simulink model "kopter_se_zavazim_simulace"  (R2024b)
settings: Solver=FixedStepAuto  StartTime=0.0  StopTime=5  FixedStep=0.01  RelTol=1e-3
values from neighbouring files (symbols this model uses):
  b_moment = 0.01    [parametry_kopter_se_zavazim.m]
  d = 1    [parametry_kopter_se_zavazim.m]
  g = 9.81    [parametry_kopter_se_zavazim.m]
  Ip = m*d^2    (= 1)    [parametry_kopter_se_zavazim.m]
  Ixx = 1.1    [parametry_kopter_se_zavazim.m]
  Iyy = 2.989    [parametry_kopter_se_zavazim.m]
  Izz = 3.978    [parametry_kopter_se_zavazim.m]
  k = 0.01    [parametry_kopter_se_zavazim.m]
  k_thrust = 0.1    [parametry_kopter_se_zavazim.m]
  L = 0.086    [parametry_kopter_se_zavazim.m]
  M = 3.3    [parametry_kopter_se_zavazim.m]
  m = 1    [parametry_kopter_se_zavazim.m]
  Us = [M*g; 0; 0; 0]    [parametry_kopter_se_zavazim.m]
  Xinit_matrix = [xyz_init; uhly_init; zavazi_init]    [parametry_kopter_se_zavazim.m]
  Xs = [0;0;0; 0;0;0; 0;0; 0;0;0; 0;0;0; 0;0]    [parametry_kopter_se_zavazim.m]
undefined symbols (not defined in the file or in its folder): Xinit_ss
libraries: simulink_extras x4
settings Model: Creator=Admin  LastModifiedBy=Admin

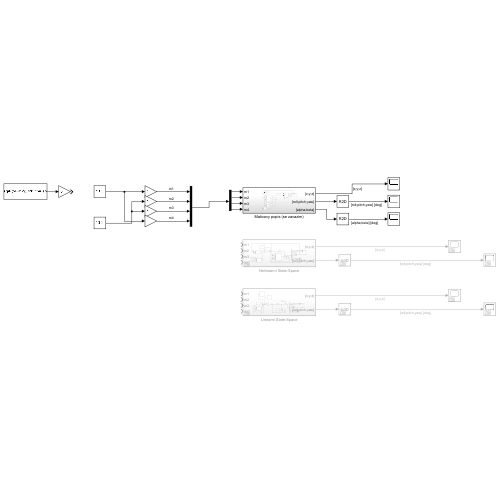
[thumbnail: Simulink's stored preview of the top-level diagram]
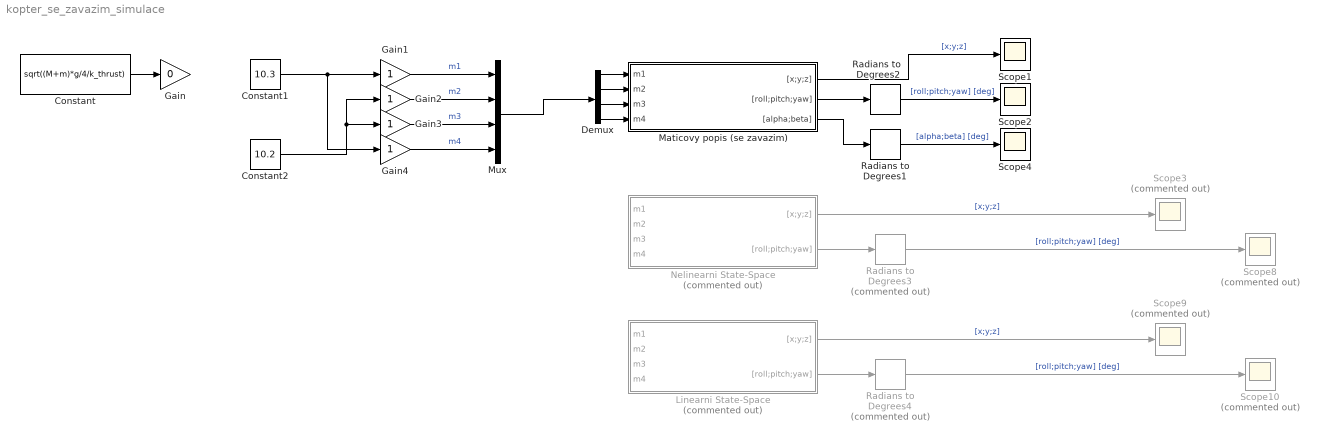
== system kopter_se_zavazim_simulace ==
  Constant : Constant  Value=sqrt((M+m)*g/4/k_thrust)
  Constant1 : Constant  Value=10.3
  Constant2 : Constant  Value=10.2
  Demux : Demux
  Gain : Gain  Gain=0
  Gain{1..4} (4 alike) : Gain
  Linearni State-Space : Subsystem  Commented=on
  Maticovy popis (se zavazim) : Subsystem
  Mux : Mux
  Nelinearni State-Space : Subsystem  Commented=on
  Radians to Degrees1 : simulink_extras/Transformations/Radians to Degrees
  Radians to Degrees2 : simulink_extras/Transformations/Radians to Degrees
  Radians to Degrees3 : simulink_extras/Transformations/Radians to Degrees  Commented=on
  Radians to Degrees4 : simulink_extras/Transformations/Radians to Degrees  Commented=on
  Scope1 : Scope
  Scope{3,8..10} (4 alike) : Scope  Commented=on
  Scope2 : Scope
  Scope4 : Scope
  wires:
  Gain4/1 -> Mux/4  "m4"
  Constant/1 -> Gain/1
  Gain1/1 -> Mux/1  "m1"
  Gain3/1 -> Mux/3  "m3"
  Gain2/1 -> Mux/2  "m2"
  Maticovy popis (se zavazim)/1("[x;y;z]") -> Scope1/1  "[x;y;z]"
  Radians to Degrees2/1 -> Scope2/1  "[roll;pitch;yaw] [deg]"
  Maticovy popis (se zavazim)/2("[roll;pitch;yaw]") -> Radians to Degrees2/1
  Radians to Degrees3/1 -> Scope8/1  "[roll;pitch;yaw] [deg]"
  Nelinearni State-Space/1("[x;y;z]") -> Scope3/1  "[x;y;z]"
  Nelinearni State-Space/2("[roll;pitch;yaw]") -> Radians to Degrees3/1
  Radians to Degrees4/1 -> Scope10/1  "[roll;pitch;yaw] [deg]"
  Linearni State-Space/2("[roll;pitch;yaw]") -> Radians to Degrees4/1
  Linearni State-Space/1("[x;y;z]") -> Scope9/1  "[x;y;z]"
  Constant1/1 -> Gain4/1, Gain1/1
  Constant2/1 -> Gain3/1, Gain2/1
  Maticovy popis (se zavazim)/3("[alpha;beta]") -> Radians to Degrees1/1
  Radians to Degrees1/1 -> Scope4/1  "[alpha;beta] [deg]"
  Demux/1 -> Maticovy popis (se zavazim)/1(m1)
  Demux/2 -> Maticovy popis (se zavazim)/2(m2)
  Demux/3 -> Maticovy popis (se zavazim)/3(m3)
  Demux/4 -> Maticovy popis (se zavazim)/4(m4)
  Mux/1 -> Demux/1

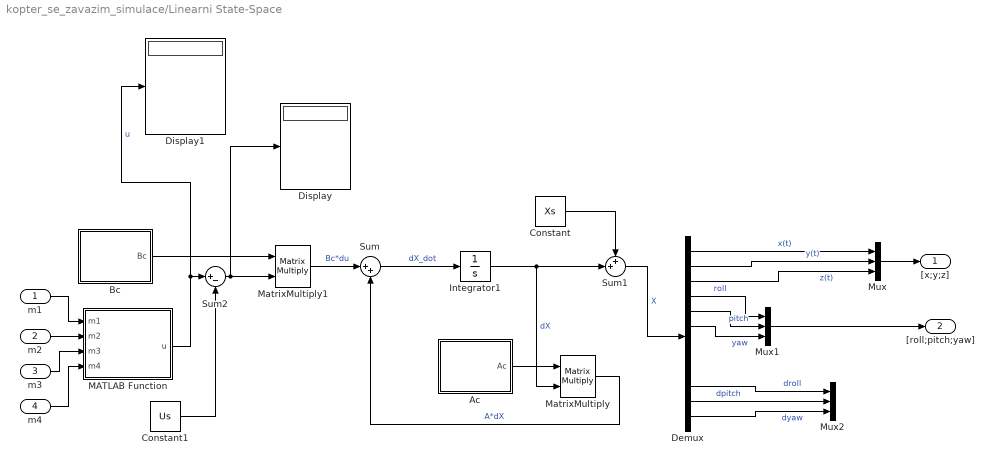
== system kopter_se_zavazim_simulace/Linearni State-Space ==
  m1 : Inport
  m2 : Inport  Port=2
  m3 : Inport  Port=3
  m4 : Inport  Port=4
  Ac : MATLAB Function  TreatAsAtomicUnit=on
  Bc : MATLAB Function  TreatAsAtomicUnit=on
  Constant : Constant  Value=Xs
  Constant1 : Constant  Value=Us
  Demux : Demux  Outputs=12
  Display : Display
  Display1 : Display
  Integrator1 : Integrator  InitialCondition=Xinit_ss
  MATLAB Function : MATLAB Function  TreatAsAtomicUnit=on
  MatrixMultiply : Product  Multiplication=Matrix(*)
  MatrixMultiply1 : Product  Multiplication=Matrix(*)
  Mux : Mux  Inputs=3
  Mux1 : Mux  Inputs=3
  Mux2 : Mux  Inputs=3
  Sum : Sum  Inputs=|++
  Sum1 : Sum  Inputs=++|
  Sum2 : Sum  Inputs=|+-
  "[x;y;z]" : Outport
  "[roll;pitch;yaw]" : Outport  Port=2
  wires:
  MATLAB Function/1(u) -> Display1/1, Sum2/1  "u"
  m3/1 -> MATLAB Function/3(m3)
  m2/1 -> MATLAB Function/2(m2)
  m4/1 -> MATLAB Function/4(m4)
  m1/1 -> MATLAB Function/1(m1)
  Ac/1(Ac) -> MatrixMultiply/1
  Integrator1/1 -> Sum1/2, MatrixMultiply/2  "dX"
  Demux/1 -> Mux/1  "x(t)"
  Demux/2 -> Mux/2  "y(t)"
  Demux/3 -> Mux/3  "z(t)"
  Mux/1 -> "[x;y;z]"/1
  Demux/4 -> Mux1/1  "roll"
  Demux/5 -> Mux1/2  "pitch"
  Demux/6 -> Mux1/3  "yaw"
  Mux1/1 -> "[roll;pitch;yaw]"/1
  Demux/10 -> Mux2/1  "droll"
  Demux/11 -> Mux2/2  "dpitch"
  Demux/12 -> Mux2/3  "dyaw"
  Sum/1 -> Integrator1/1  "dX_dot"
  MatrixMultiply1/1 -> Sum/1  "Bc*du"
  MatrixMultiply/1 -> Sum/2  "A*dX"
  Bc/1(Bc) -> MatrixMultiply1/1
  Sum1/1 -> Demux/1  "X"
  Constant/1 -> Sum1/1
  Constant1/1 -> Sum2/2
  Sum2/1 -> Display/1, MatrixMultiply1/2

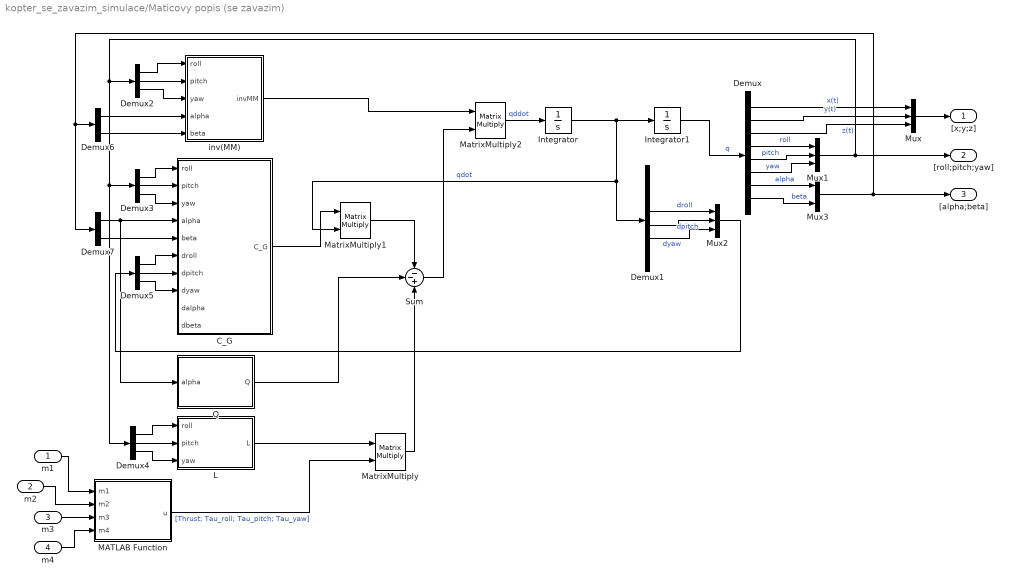
== system kopter_se_zavazim_simulace/Maticovy popis (se zavazim) ==
  m1 : Inport
  m2 : Inport  Port=2
  m3 : Inport  Port=3
  m4 : Inport  Port=4
  C_G : MATLAB Function  TreatAsAtomicUnit=on
  Demux : Demux  Outputs=8
  Demux1 : Demux  Outputs=8
  Demux{2..5} (4 alike) : Demux  Outputs=3
  Demux6 : Demux  Outputs=2
  Demux7 : Demux  Outputs=2
  Integrator : Integrator  InitialCondition=[0;0;0;0;0;0;0;0]
  Integrator1 : Integrator  InitialCondition=Xinit_matrix
  L : MATLAB Function  TreatAsAtomicUnit=on
  MATLAB Function : MATLAB Function  TreatAsAtomicUnit=on
  MatrixMultiply : Product  Multiplication=Matrix(*)
  MatrixMultiply1 : Product  Multiplication=Matrix(*)
  MatrixMultiply2 : Product  Multiplication=Matrix(*)
  Mux : Mux  Inputs=3
  Mux1 : Mux  Inputs=3
  Mux2 : Mux  Inputs=3
  Mux3 : Mux  Inputs=2
  Q : MATLAB Function  TreatAsAtomicUnit=on
  Sum : Sum  Inputs=--+
  inv(MM) : MATLAB Function  TreatAsAtomicUnit=on
  "[x;y;z]" : Outport
  "[roll;pitch;yaw]" : Outport  Port=2
  "[alpha;beta]" : Outport  Port=3
  wires:
  inv(MM)/1(invMM) -> MatrixMultiply2/1
  L/1(L) -> MatrixMultiply/1
  MATLAB Function/1(u) -> MatrixMultiply/2  "[Thrust; Tau_roll; Tau_pitch; Tau_yaw]"
  m3/1 -> MATLAB Function/3(m3)
  m2/1 -> MATLAB Function/2(m2)
  m4/1 -> MATLAB Function/4(m4)
  MatrixMultiply/1 -> Sum/3
  m1/1 -> MATLAB Function/1(m1)
  Q/1(Q) -> Sum/2
  C_G/1(C_G) -> MatrixMultiply1/1
  MatrixMultiply1/1 -> Sum/1
  Sum/1 -> MatrixMultiply2/2
  MatrixMultiply2/1 -> Integrator/1  "qddot"
  Integrator/1 -> MatrixMultiply1/2, Demux1/1, Integrator1/1  "qdot"
  Integrator1/1 -> Demux/1  "q"
  Demux/1 -> Mux/1  "x(t)"
  Demux/2 -> Mux/2  "y(t)"
  Demux/3 -> Mux/3  "z(t)"
  Mux/1 -> "[x;y;z]"/1
  Demux/4 -> Mux1/1  "roll"
  Demux/5 -> Mux1/2  "pitch"
  Demux/6 -> Mux1/3  "yaw"
  Mux1/1 -> "[roll;pitch;yaw]"/1, Demux4/1, Demux3/1, Demux2/1
  Demux1/4 -> Mux2/1  "droll"
  Demux1/5 -> Mux2/2  "dpitch"
  Demux1/6 -> Mux2/3  "dyaw"
  Demux2/1 -> inv(MM)/1(roll)
  Demux2/2 -> inv(MM)/2(pitch)
  Demux2/3 -> inv(MM)/3(yaw)
  Demux3/2 -> C_G/2(pitch)
  Demux3/1 -> C_G/1(roll)
  Demux3/3 -> C_G/3(yaw)
  Demux4/2 -> L/2(pitch)
  Demux4/1 -> L/1(roll)
  Demux4/3 -> L/3(yaw)
  Demux5/2 -> C_G/7(dpitch)
  Demux5/1 -> C_G/6(droll)
  Demux5/3 -> C_G/8(dyaw)
  Mux2/1 -> Demux5/1
  Demux/7 -> Mux3/1  "alpha"
  Demux/8 -> Mux3/2  "beta"
  Mux3/1 -> Demux7/1, Demux6/1, "[alpha;beta]"/1
  Demux6/1 -> inv(MM)/4(alpha)
  Demux6/2 -> inv(MM)/5(beta)
  Demux7/2 -> C_G/5(beta)
  Demux7/1 -> Q/1(alpha), C_G/4(alpha)

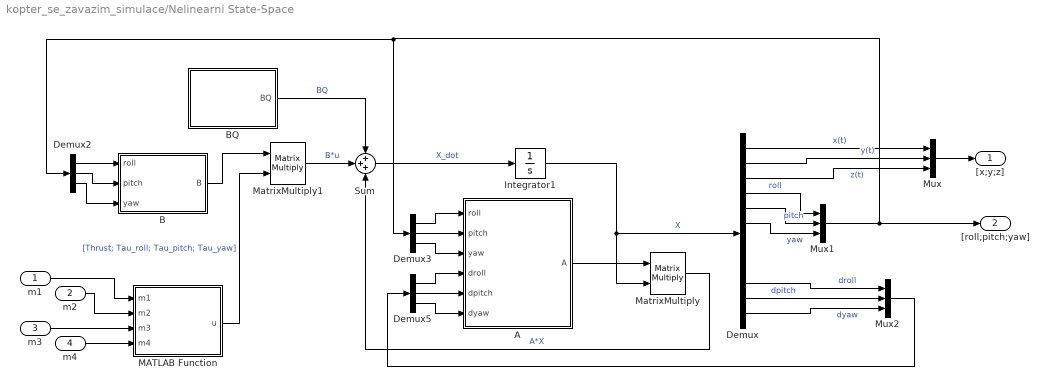
== system kopter_se_zavazim_simulace/Nelinearni State-Space ==
  m1 : Inport
  m2 : Inport  Port=2
  m3 : Inport  Port=3
  m4 : Inport  Port=4
  A : MATLAB Function  TreatAsAtomicUnit=on
  B : MATLAB Function  TreatAsAtomicUnit=on
  BQ : MATLAB Function  TreatAsAtomicUnit=on
  Demux : Demux  Outputs=12
  Demux2 : Demux  Outputs=3
  Demux3 : Demux  Outputs=3
  Demux5 : Demux  Outputs=3
  Integrator1 : Integrator  InitialCondition=Xinit_ss
  MATLAB Function : MATLAB Function  TreatAsAtomicUnit=on
  MatrixMultiply : Product  Multiplication=Matrix(*)
  MatrixMultiply1 : Product  Multiplication=Matrix(*)
  Mux : Mux  Inputs=3
  Mux1 : Mux  Inputs=3
  Mux2 : Mux  Inputs=3
  Sum : Sum  Inputs=+++
  "[x;y;z]" : Outport
  "[roll;pitch;yaw]" : Outport  Port=2
  wires:
  MATLAB Function/1(u) -> MatrixMultiply1/2  "[Thrust; Tau_roll; Tau_pitch; Tau_yaw]"
  m3/1 -> MATLAB Function/3(m3)
  m2/1 -> MATLAB Function/2(m2)
  m4/1 -> MATLAB Function/4(m4)
  m1/1 -> MATLAB Function/1(m1)
  A/1(A) -> MatrixMultiply/1
  Integrator1/1 -> Demux/1, MatrixMultiply/2  "X"
  Demux/1 -> Mux/1  "x(t)"
  Demux/2 -> Mux/2  "y(t)"
  Demux/3 -> Mux/3  "z(t)"
  Mux/1 -> "[x;y;z]"/1
  Demux/4 -> Mux1/1  "roll"
  Demux/5 -> Mux1/2  "pitch"
  Demux/6 -> Mux1/3  "yaw"
  Mux1/1 -> Demux2/1, Demux3/1, "[roll;pitch;yaw]"/1
  Demux/10 -> Mux2/1  "droll"
  Demux/11 -> Mux2/2  "dpitch"
  Demux/12 -> Mux2/3  "dyaw"
  Demux2/1 -> B/1(roll)
  Demux2/2 -> B/2(pitch)
  Demux2/3 -> B/3(yaw)
  Demux3/2 -> A/2(pitch)
  Demux3/1 -> A/1(roll)
  Demux3/3 -> A/3(yaw)
  Demux5/2 -> A/5(dpitch)
  Demux5/1 -> A/4(droll)
  Demux5/3 -> A/6(dyaw)
  Sum/1 -> Integrator1/1  "X_dot"
  BQ/1(BQ) -> Sum/1  "BQ"
  MatrixMultiply1/1 -> Sum/2  "B*u"
  B/1(B) -> MatrixMultiply1/1
  MatrixMultiply/1 -> Sum/3  "A*X"
  Mux2/1 -> Demux5/1

== matlab function kopter_se_zavazim_simulace/Nelinearni State-Space/BQ ==
  data: BQ output; g parameter
function BQ = fcn(g)
% Matice vstupu tihy
BQ = [0 0 0 0 0 0 0 0 -g 0 0 0]';

== matlab function kopter_se_zavazim_simulace/Nelinearni State-Space/MATLAB Function ==
  data: u output; m1 input; m2 input; m3 input; m4 input; k_thrust parameter; b_moment parameter; L parameter
function u = fcn(m1, m2, m3, m4, k_thrust, b_moment, L)

Thrust = k_thrust*(m1^2 + m2^2 + m3^2 + m4^2);
Tau_roll = L*k_thrust*(m1^2 + m4^2 - m2^2 - m3^2);
Tau_pitch = L*k_thrust*(m4^2 + m3^2 - m1^2 - m2^2);
Tau_yaw = b_moment*(m1^2 + m3^2 - m2^2 - m4^2);

u = [Thrust; Tau_roll; Tau_pitch; Tau_yaw];

== matlab function kopter_se_zavazim_simulace/Linearni State-Space/Bc ==
  data: M parameter; Bc output; Ixx parameter; Iyy parameter; Izz parameter
function Bc = fcn(M, Ixx, Iyy, Izz)
% Matice Ac linearizovana

Bc = [
  0,     0,     0,     0;
  0,     0,     0,     0;
  0,     0,     0,     0;
  0,     0,     0,     0;
  0,     0,     0,     0;
  0,     0,     0,     0;
  0,     0,     0,     0;
  0,     0,     0,     0;
1/M,     0,     0,     0;
  0, 1/Ixx,     0,     0;
  0,     0, 1/Iyy,     0;
  0,     0,     0, 1/Izz];

== matlab function kopter_se_zavazim_simulace/Nelinearni State-Space/B ==
  data: roll input; B output; pitch input; yaw input; M parameter; Ixx parameter; Iyy parameter; Izz parameter
function B = fcn(roll, pitch, yaw, M, Ixx, Iyy, Izz)
% Matice vstupu do soustavy kvadrokoptery

phi_t = roll;
theta_t = pitch;
psi_t = yaw;

B = [
                                                              0,     0,                                                                          0,                                                                          0;
                                                              0,     0,                                                                          0,                                                                          0;
                                                              0,     0,                                                                          0,                                                                          0;
                                                              0,     0,                                                                          0,                                                                          0;
                                                              0,     0,                                                                          0,                                                                          0;
                                                              0,     0,                                                                          0,                                                                          0;
 (sin(phi_t)*sin(psi_t) + cos(phi_t)*cos(psi_t)*sin(theta_t))/M,     0,                                                                          0,                                                                          0;
-(cos(psi_t)*sin(phi_t) - cos(phi_t)*sin(psi_t)*sin(theta_t))/M,     0,                                                                          0,                                                                          0;
                                    (cos(phi_t)*cos(theta_t))/M,     0,                                                                          0,                                                                          0;
                                                              0, 1/Ixx, (sin(phi_t)*sin(theta_t))/(Iyy*cos(theta_t)*(cos(phi_t)^2 + sin(phi_t)^2)), (cos(phi_t)*sin(theta_t))/(Izz*cos(theta_t)*(cos(phi_t)^2 + sin(phi_t)^2));
                                                              0,     0,                             cos(phi_t)/(Iyy*(cos(phi_t)^2 + sin(phi_t)^2)),                            -sin(phi_t)/(Izz*(cos(phi_t)^2 + sin(phi_t)^2));
                                                              0,     0,                sin(phi_t)/(Iyy*cos(theta_t)*(cos(phi_t)^2 + sin(phi_t)^2)),                cos(phi_t)/(Izz*cos(theta_t)*(cos(phi_t)^2 + sin(phi_t)^2))];

== matlab function kopter_se_zavazim_simulace/Linearni State-Space/MATLAB Function ==
  data: u output; m1 input; m2 input; m3 input; m4 input; k_thrust parameter; b_moment parameter; L parameter
function u = fcn(m1, m2, m3, m4, k_thrust, b_moment, L)

Thrust = k_thrust*(m1^2 + m2^2 + m3^2 + m4^2);
Tau_roll = L*k_thrust*(m1^2 + m4^2 - m2^2 - m3^2);
Tau_pitch = L*k_thrust*(m4^2 + m3^2 - m1^2 - m2^2);
Tau_yaw = b_moment*(m1^2 + m3^2 - m2^2 - m4^2);

u = [Thrust; Tau_roll; Tau_pitch; Tau_yaw];

== matlab function kopter_se_zavazim_simulace/Linearni State-Space/Ac ==
  data: Ac output; k parameter; g parameter; M parameter
function Ac = fcn(k, g, M)
% Matice Ac linearizovana

Ac = [ 
0, 0, 0,  0, 0, 0,    1,    0,    0, 0, 0, 0;
0, 0, 0,  0, 0, 0,    0,    1,    0, 0, 0, 0;
0, 0, 0,  0, 0, 0,    0,    0,    1, 0, 0, 0;
0, 0, 0,  0, 0, 0,    0,    0,    0, 1, 0, 0;
0, 0, 0,  0, 0, 0,    0,    0,    0, 0, 1, 0;
0, 0, 0,  0, 0, 0,    0,    0,    0, 0, 0, 1;
0, 0, 0,  0, g, 0, -k/M,    0,    0, 0, 0, 0;
0, 0, 0, -g, 0, 0,    0, -k/M,    0, 0, 0, 0;
0, 0, 0,  0, 0, 0,    0,    0, -k/M, 0, 0, 0;
0, 0, 0,  0, 0, 0,    0,    0,    0, 0, 0, 0;
0, 0, 0,  0, 0, 0,    0,    0,    0, 0, 0, 0;
0, 0, 0,  0, 0, 0,    0,    0,    0, 0, 0, 0];

== matlab function kopter_se_zavazim_simulace/Maticovy popis (se zavazim)/C_G ==
  data: roll input; C_G output; pitch input; yaw input; alpha input; beta input; droll input; dpitch input; dyaw input; dalpha input; dbeta input; Ixx parameter; Iyy parameter; Izz parameter; d parameter; m parameter
function C_G = fcn(roll, pitch, yaw, alpha, beta, droll, dpitch, dyaw, dalpha, dbeta, Ixx, Iyy, Izz, d, m)
% Matice Coriolisovych sil a odporu vzduchu

phi_t = roll;
theta_t = pitch;
psi_t = yaw;

phi_dot_t = droll;
theta_dot_t = dpitch;
psi_dot_t = dyaw;

alpha_t = alpha;
beta_t = beta;

alpha_dot_t = dalpha;
beta_dot_t = dbeta;


C_G = [
0, 0, 0,                                                                                                                                                                                                                                                                    0,                                                                                                                                                                                                                                           0,                                                                                                                                   0,                                                         - alpha_dot_t*d*m*cos(beta_t)*sin(alpha_t) - 2*beta_dot_t*d*m*cos(alpha_t)*sin(beta_t),                                                                    -beta_dot_t*d*m*cos(beta_t)*sin(alpha_t);
0, 0, 0,                                                                                                                                                                                                                                                                    0,                                                                                                                                                                                                                                           0,                                                                                                                                   0,                                                           2*beta_dot_t*d*m*cos(alpha_t)*cos(beta_t) - alpha_dot_t*d*m*sin(alpha_t)*sin(beta_t),                                                                    -beta_dot_t*d*m*sin(alpha_t)*sin(beta_t);
0, 0, 0,                                                                                                                                                                                                                                                                    0,                                                                                                                                                                                                                                           0,                                                                                                                                   0,                                                                                                                   alpha_dot_t*d*m*cos(alpha_t),                                                                                                           0;
0, 0, 0,                                                                                                                                                                                                                                                                    0,          theta_dot_t*(Iyy*cos(phi_t)*sin(phi_t) - Izz*cos(phi_t)*sin(phi_t)) - psi_dot_t*(Ixx*cos(theta_t) + Iyy*cos(phi_t)^2*cos(theta_t) - Izz*cos(phi_t)^2*cos(theta_t) - Iyy*cos(theta_t)*sin(phi_t)^2 + Izz*cos(theta_t)*sin(phi_t)^2),                                    -psi_dot_t*(Iyy*cos(phi_t)*cos(theta_t)^2*sin(phi_t) - Izz*cos(phi_t)*cos(theta_t)^2*sin(phi_t)),                                                                                                                                              0,                                                                                                           0;
0, 0, 0,                               psi_dot_t*(Ixx*cos(theta_t) + Iyy*cos(phi_t)^2*cos(theta_t) - Izz*cos(phi_t)^2*cos(theta_t) - Iyy*cos(theta_t)*sin(phi_t)^2 + Izz*cos(theta_t)*sin(phi_t)^2) - theta_dot_t*(2*Iyy*cos(phi_t)*sin(phi_t) - 2*Izz*cos(phi_t)*sin(phi_t)),                                                                                                                                                                                                                                           0, psi_dot_t*(Izz*cos(phi_t)^2*cos(theta_t)*sin(theta_t) - Ixx*cos(theta_t)*sin(theta_t) + Iyy*cos(theta_t)*sin(phi_t)^2*sin(theta_t)),                                                                                                                                              0,                                                                                                           0;
0, 0, 0, psi_dot_t*(2*Iyy*cos(phi_t)*cos(theta_t)^2*sin(phi_t) - 2*Izz*cos(phi_t)*cos(theta_t)^2*sin(phi_t)) - theta_dot_t*(Ixx*cos(theta_t) - Iyy*cos(phi_t)^2*cos(theta_t) + Izz*cos(phi_t)^2*cos(theta_t) + Iyy*cos(theta_t)*sin(phi_t)^2 - Izz*cos(theta_t)*sin(phi_t)^2), - theta_dot_t*(Iyy*cos(phi_t)*sin(phi_t)*sin(theta_t) - Izz*cos(phi_t)*sin(phi_t)*sin(theta_t)) - psi_dot_t*(2*Izz*cos(phi_t)^2*cos(theta_t)*sin(theta_t) - 2*Ixx*cos(theta_t)*sin(theta_t) + 2*Iyy*cos(theta_t)*sin(phi_t)^2*sin(theta_t)),                                                                                                                                   0,                                                                                                                                              0,                                                                                                           0;
0, 0, 0,                                                                                                                                                                                                                                                                    0,                                                                                                                                                                                                                                           0,                                                                                                                                   0, -alpha_dot_t*(d^2*m*cos(alpha_t)*cos(beta_t)^2*sin(alpha_t) - d^2*m*cos(alpha_t)*sin(alpha_t) + d^2*m*cos(alpha_t)*sin(alpha_t)*sin(beta_t)^2), -beta_dot_t*(m*cos(alpha_t)*sin(alpha_t)*d^2*cos(beta_t)^2 + m*cos(alpha_t)*sin(alpha_t)*d^2*sin(beta_t)^2);
0, 0, 0,                                                                                                                                                                                                                                                                    0,                                                                                                                                                                                                                                           0,                                                                                                                                   0,                                 beta_dot_t*(2*d^2*m*cos(alpha_t)*cos(beta_t)^2*sin(alpha_t) + 2*d^2*m*cos(alpha_t)*sin(alpha_t)*sin(beta_t)^2),                                                                                                           0];

== matlab function kopter_se_zavazim_simulace/Maticovy popis (se zavazim)/inv(MM) ==
  data: roll input; invMM output; pitch input; yaw input; alpha input; beta input; M parameter; Ixx parameter; Iyy parameter; Izz parameter; d parameter; m parameter; Ip parameter
function invMM = fcn(roll, pitch, yaw, alpha, beta, M, Ixx, Iyy, Izz, d, m, Ip)
% Matice hmotnosti a setrvacnosti

phi_t = roll;
theta_t = pitch;
psi_t = yaw;

alpha_t = alpha;
beta_t = beta;

MM = [
                        M + m,                            0,                0,                 0,                                              0,                                                                                      0, d*m*cos(alpha_t)*cos(beta_t), -d*m*sin(alpha_t)*sin(beta_t);
                            0,                        M + m,                0,                 0,                                              0,                                                                                      0, d*m*cos(alpha_t)*sin(beta_t),  d*m*cos(beta_t)*sin(alpha_t);
                            0,                            0,            M + m,                 0,                                              0,                                                                                      0,             d*m*sin(alpha_t),                             0;
                            0,                            0,                0,               Ixx,                                              0,                                                                      -Ixx*sin(theta_t),                            0,                             0;
                            0,                            0,                0,                 0,      Iyy - Iyy*sin(phi_t)^2 + Izz*sin(phi_t)^2,                                         cos(phi_t)*cos(theta_t)*sin(phi_t)*(Iyy - Izz),                            0,                             0;
                            0,                            0,                0, -Ixx*sin(theta_t), cos(phi_t)*cos(theta_t)*sin(phi_t)*(Iyy - Izz), Izz*cos(phi_t)^2*cos(theta_t)^2 + Iyy*cos(theta_t)^2*sin(phi_t)^2 + Ixx*sin(theta_t)^2,                            0,                             0;
 d*m*cos(alpha_t)*cos(beta_t), d*m*cos(alpha_t)*sin(beta_t), d*m*sin(alpha_t),                 0,                                              0,                                                                                      0,                   m*d^2 + Ip,                             0;
-d*m*sin(alpha_t)*sin(beta_t), d*m*cos(beta_t)*sin(alpha_t),                0,                 0,                                              0,                                                                                      0,                            0,     m*d^2*sin(alpha_t)^2 + Ip];
 

invMM = inv(MM);

== matlab function kopter_se_zavazim_simulace/Maticovy popis (se zavazim)/Q ==
  data: alpha input; M parameter; Q output; g parameter; m parameter; d parameter
function Q = fcn(alpha, M, g, m, d)
alpha_t = alpha;
% Matice tihovych sil
Q = [0 0 (M+m)*g 0 0 0 d*g*m*sin(alpha_t) 0]';

== matlab function kopter_se_zavazim_simulace/Maticovy popis (se zavazim)/L ==
  data: roll input; L output; pitch input; yaw input
function L = fcn(roll, pitch, yaw)
% Matice vah vstupu

phi_t = roll;
theta_t = pitch;
psi_t = yaw;

L = [
sin(phi_t)*sin(psi_t) + cos(phi_t)*cos(psi_t)*sin(theta_t), 0, 0, 0;
cos(phi_t)*sin(psi_t)*sin(theta_t) - cos(psi_t)*sin(phi_t), 0, 0, 0;
                                   cos(phi_t)*cos(theta_t), 0, 0, 0;
                                                         0, 1, 0, 0;
                                                         0, 0, 1, 0;
                                                         0, 0, 0, 1;
                                                         0, 0, 0, 0;
                                                         0, 0, 0, 0];

== matlab function kopter_se_zavazim_simulace/Maticovy popis (se zavazim)/MATLAB Function ==
  data: u output; m1 input; m2 input; m3 input; m4 input; k_thrust parameter; b_moment parameter; L parameter
function u = fcn(m1, m2, m3, m4, k_thrust, b_moment, L)

Thrust = k_thrust*(m1^2 + m2^2 + m3^2 + m4^2);
Tau_roll = L*k_thrust*(m1^2 + m4^2 - m2^2 - m3^2);
Tau_pitch = L*k_thrust*(m4^2 + m3^2 - m1^2 - m2^2);
Tau_yaw = b_moment*(m1^2 + m3^2 - m2^2 - m4^2);

u = [Thrust; Tau_roll; Tau_pitch; Tau_yaw];

== matlab function kopter_se_zavazim_simulace/Nelinearni State-Space/A ==
  data: roll input; A output; pitch input; yaw input; droll input; dpitch input; dyaw input; k parameter; Ixx parameter; Iyy parameter; Izz parameter; M parameter
function A = fcn(roll, pitch, yaw, droll, dpitch, dyaw, k, Ixx, Iyy, Izz, M)
% Matice dynamiky A

phi_t = roll;
theta_t = pitch;
psi_t = yaw;

phi_dot_t = droll;
theta_dot_t = dpitch;
psi_dot_t = dyaw;

A = [
0, 0, 0, 0, 0, 0,    1,    0,    0,                                                                                                                                                                                                                                                                                                                                                                                                                                                                                                                               0,                                                                                                                                                                                                                                                                                                                                                                                                                                                                                                                                                                                                                                    0,                                                                                                                                                                                                                                                                                                                                                                                                                                                                                         0;
0, 0, 0, 0, 0, 0,    0,    1,    0,                                                                                                                                                                                                                                                                                                                                                                                                                                                                                                                               0,                                                                                                                                                                                                                                                                                                                                                                                                                                                                                                                                                                                                                                    0,                                                                                                                                                                                                                                                                                                                                                                                                                                                                                         0;
0, 0, 0, 0, 0, 0,    0,    0,    1,                                                                                                                                                                                                                                                                                                                                                                                                                                                                                                                               0,                                                                                                                                                                                                                                                                                                                                                                                                                                                                                                                                                                                                                                    0,                                                                                                                                                                                                                                                                                                                                                                                                                                                                                         0;
0, 0, 0, 0, 0, 0,    0,    0,    0,                                                                                                                                                                                                                                                                                                                                                                                                                                                                                                                               1,                                                                                                                                                                                                                                                                                                                                                                                                                                                                                                                                                                                                                                    0,                                                                                                                                                                                                                                                                                                                                                                                                                                                                                         0;
0, 0, 0, 0, 0, 0,    0,    0,    0,                                                                                                                                                                                                                                                                                                                                                                                                                                                                                                                               0,                                                                                                                                                                                                                                                                                                                                                                                                                                                                                                                                                                                                                                    1,                                                                                                                                                                                                                                                                                                                                                                                                                                                                                         0;
0, 0, 0, 0, 0, 0,    0,    0,    0,                                                                                                                                                                                                                                                                                                                                                                                                                                                                                                                               0,                                                                                                                                                                                                                                                                                                                                                                                                                                                                                                                                                                                                                                    0,                                                                                                                                                                                                                                                                                                                                                                                                                                                                                         1;
0, 0, 0, 0, 0, 0, -k/M,    0,    0,                                                                                                                                                                                                                                                                                                                                                                                                                                                                                                                               0,                                                                                                                                                                                                                                                                                                                                                                                                                                                                                                                                                                                                                                    0,                                                                                                                                                                                                                                                                                                                                                                                                                                                                                         0;
0, 0, 0, 0, 0, 0,    0, -k/M,    0,                                                                                                                                                                                                                                                                                                                                                                                                                                                                                                                               0,                                                                                                                                                                                                                                                                                                                                                                                                                                                                                                                                                                                                                                    0,                                                                                                                                                                                                                                                                                                                                                                                                                                                                                         0;
0, 0, 0, 0, 0, 0,    0,    0, -k/M,                                                                                                                                                                                                                                                                                                                                                                                                                                                                                                                               0,                                                                                                                                                                                                                                                                                                                                                                                                                                                                                                                                                                                                                                    0,                                                                                                                                                                                                                                                                                                                                                                                                                                                                                         0;
0, 0, 0, 0, 0, 0,    0,    0,    0, (cos(phi_t)*sin(theta_t)*(psi_dot_t*(Ixx*cos(theta_t)*sin(phi_t) - Iyy*cos(theta_t)*sin(phi_t) + Izz*cos(theta_t)*sin(phi_t)) + theta_dot_t*(Ixx*cos(phi_t) - Iyy*cos(phi_t) + Izz*cos(phi_t))))/(Izz*(cos(theta_t)*cos(phi_t)^2 + cos(theta_t)*sin(phi_t)^2)) - (sin(phi_t)*sin(theta_t)*(psi_dot_t*(Ixx*cos(phi_t)*cos(theta_t) + Iyy*cos(phi_t)*cos(theta_t) - Izz*cos(phi_t)*cos(theta_t)) - theta_dot_t*(Ixx*sin(phi_t) + Iyy*sin(phi_t) - Izz*sin(phi_t))))/(Iyy*(cos(theta_t)*cos(phi_t)^2 + cos(theta_t)*sin(phi_t)^2)), (psi_dot_t*(Ixx*cos(theta_t) + Iyy*cos(phi_t)^2*cos(theta_t) - Izz*cos(phi_t)^2*cos(theta_t) - Iyy*cos(theta_t)*sin(phi_t)^2 + Izz*cos(theta_t)*sin(phi_t)^2) - theta_dot_t*(Iyy*cos(phi_t)*sin(phi_t) - Izz*cos(phi_t)*sin(phi_t)))/Ixx + (psi_dot_t*cos(phi_t)*sin(theta_t)*(Iyy*cos(phi_t)*sin(theta_t) - Ixx*cos(phi_t)*sin(theta_t) + Izz*cos(phi_t)*sin(theta_t)))/(Izz*(cos(theta_t)*cos(phi_t)^2 + cos(theta_t)*sin(phi_t)^2)) + (psi_dot_t*sin(phi_t)*sin(theta_t)*(Iyy*sin(phi_t)*sin(theta_t) - Ixx*sin(phi_t)*sin(theta_t) + Izz*sin(phi_t)*sin(theta_t)))/(Iyy*(cos(theta_t)*cos(phi_t)^2 + cos(theta_t)*sin(phi_t)^2)), (psi_dot_t*(Iyy*cos(phi_t)*cos(theta_t)^2*sin(phi_t) - Izz*cos(phi_t)*cos(theta_t)^2*sin(phi_t)))/Ixx + (psi_dot_t*sin(phi_t)*sin(theta_t)*(Ixx*cos(phi_t)*cos(theta_t)*sin(theta_t) - Izz*cos(phi_t)*cos(theta_t)*sin(theta_t)))/(Iyy*(cos(theta_t)*cos(phi_t)^2 + cos(theta_t)*sin(phi_t)^2)) - (psi_dot_t*cos(phi_t)*sin(theta_t)*(Ixx*cos(theta_t)*sin(phi_t)*sin(theta_t) - Iyy*cos(theta_t)*sin(phi_t)*sin(theta_t)))/(Izz*(cos(theta_t)*cos(phi_t)^2 + cos(theta_t)*sin(phi_t)^2));
0, 0, 0, 0, 0, 0,    0,    0,    0,                                                                             - (cos(phi_t)*(psi_dot_t*(Ixx*cos(phi_t)*cos(theta_t) + Iyy*cos(phi_t)*cos(theta_t) - Izz*cos(phi_t)*cos(theta_t)) - theta_dot_t*(Ixx*sin(phi_t) + Iyy*sin(phi_t) - Izz*sin(phi_t))))/(Iyy*(cos(phi_t)^2 + sin(phi_t)^2)) - (sin(phi_t)*(psi_dot_t*(Ixx*cos(theta_t)*sin(phi_t) - Iyy*cos(theta_t)*sin(phi_t) + Izz*cos(theta_t)*sin(phi_t)) + theta_dot_t*(Ixx*cos(phi_t) - Iyy*cos(phi_t) + Izz*cos(phi_t))))/(Izz*(cos(phi_t)^2 + sin(phi_t)^2)),                                                                                                                                                                                                                                                                                                                          (psi_dot_t*cos(phi_t)*(Iyy*sin(phi_t)*sin(theta_t) - Ixx*sin(phi_t)*sin(theta_t) + Izz*sin(phi_t)*sin(theta_t)))/(Iyy*(cos(phi_t)^2 + sin(phi_t)^2)) - (psi_dot_t*sin(phi_t)*(Iyy*cos(phi_t)*sin(theta_t) - Ixx*cos(phi_t)*sin(theta_t) + Izz*cos(phi_t)*sin(theta_t)))/(Izz*(cos(phi_t)^2 + sin(phi_t)^2)),                                                                                                                                                                                       (psi_dot_t*cos(phi_t)*(Ixx*cos(phi_t)*cos(theta_t)*sin(theta_t) - Izz*cos(phi_t)*cos(theta_t)*sin(theta_t)))/(Iyy*(cos(phi_t)^2 + sin(phi_t)^2)) + (psi_dot_t*sin(phi_t)*(Ixx*cos(theta_t)*sin(phi_t)*sin(theta_t) - Iyy*cos(theta_t)*sin(phi_t)*sin(theta_t)))/(Izz*(cos(phi_t)^2 + sin(phi_t)^2));
0, 0, 0, 0, 0, 0,    0,    0,    0,                           (cos(phi_t)*(psi_dot_t*(Ixx*cos(theta_t)*sin(phi_t) - Iyy*cos(theta_t)*sin(phi_t) + Izz*cos(theta_t)*sin(phi_t)) + theta_dot_t*(Ixx*cos(phi_t) - Iyy*cos(phi_t) + Izz*cos(phi_t))))/(Izz*(cos(theta_t)*cos(phi_t)^2 + cos(theta_t)*sin(phi_t)^2)) - (sin(phi_t)*(psi_dot_t*(Ixx*cos(phi_t)*cos(theta_t) + Iyy*cos(phi_t)*cos(theta_t) - Izz*cos(phi_t)*cos(theta_t)) - theta_dot_t*(Ixx*sin(phi_t) + Iyy*sin(phi_t) - Izz*sin(phi_t))))/(Iyy*(cos(theta_t)*cos(phi_t)^2 + cos(theta_t)*sin(phi_t)^2)),                                                                                                                                                                                                                                                                      (psi_dot_t*cos(phi_t)*(Iyy*cos(phi_t)*sin(theta_t) - Ixx*cos(phi_t)*sin(theta_t) + Izz*cos(phi_t)*sin(theta_t)))/(Izz*(cos(theta_t)*cos(phi_t)^2 + cos(theta_t)*sin(phi_t)^2)) + (psi_dot_t*sin(phi_t)*(Iyy*sin(phi_t)*sin(theta_t) - Ixx*sin(phi_t)*sin(theta_t) + Izz*sin(phi_t)*sin(theta_t)))/(Iyy*(cos(theta_t)*cos(phi_t)^2 + cos(theta_t)*sin(phi_t)^2)),                                                                                                                                   (psi_dot_t*sin(phi_t)*(Ixx*cos(phi_t)*cos(theta_t)*sin(theta_t) - Izz*cos(phi_t)*cos(theta_t)*sin(theta_t)))/(Iyy*(cos(theta_t)*cos(phi_t)^2 + cos(theta_t)*sin(phi_t)^2)) - (psi_dot_t*cos(phi_t)*(Ixx*cos(theta_t)*sin(phi_t)*sin(theta_t) - Iyy*cos(theta_t)*sin(phi_t)*sin(theta_t)))/(Izz*(cos(theta_t)*cos(phi_t)^2 + cos(theta_t)*sin(phi_t)^2))];
